simulink model "SistemaNL"  (R2026a)
settings: Solver=VariableStepAuto
settings Model: Creator=admin  LastModifiedBy=admin

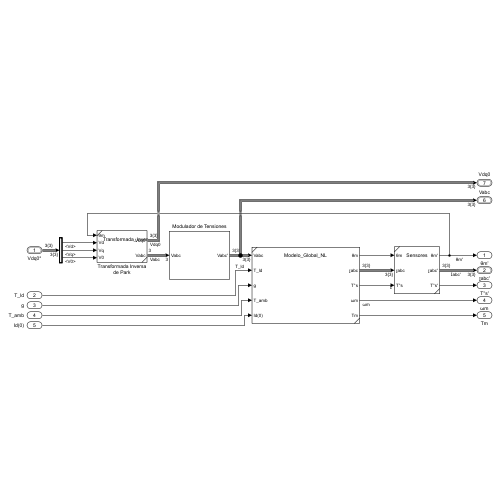
[thumbnail: Simulink's stored preview of the top-level diagram]
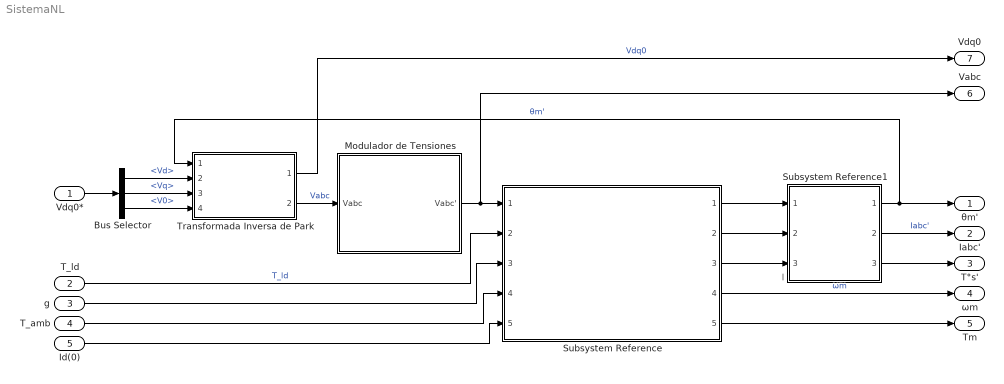
== system SistemaNL ==
  note: Ⅰ
  Vdq0* : Inport  OutDataTypeStr=Bus: Vdq0
  T_ld : Inport  Port=2
  g : Inport  Port=3
  T_amb : Inport  Port=4
  Id(0) : Inport  Port=5
  Bus Selector : BusSelector  OutputSignals=Vd,Vq,V0
  Modulador de Tensiones : Subsystem
  Subsystem Reference : Subsystem  ReferencedSubsystem=Modelo_Global_NL
  Subsystem Reference1 : Subsystem  ReferencedSubsystem=Sensores
  Transformada Inversa de Park : Subsystem  ReferencedSubsystem=Transformada_Inversa_de_Park_V
  θm' : Outport
  Ⅰabc' : Outport  Port=2  OutDataTypeStr=Bus: Iabc
  T°s' : Outport  Port=3
  ωm : Outport  Port=4
  Tm : Outport  Port=5
  Vabc : Outport  Port=6  OutDataTypeStr=Bus: Vabc
  Vdq0 : Outport  Port=7  OutDataTypeStr=Bus: Vdq0
  wires:
  Subsystem Reference1/2 -> Ⅰabc'/1  "Ⅰabc'"
  Subsystem Reference1/1 -> Transformada Inversa de Park/1, θm'/1  "θm'"
  Subsystem Reference1/3 -> T°s'/1
  Subsystem Reference/5 -> Tm/1
  Subsystem Reference/2 -> Subsystem Reference1/2
  g/1 -> Subsystem Reference/3
  Modulador de Tensiones/1(Vabc') -> Vabc/1, Subsystem Reference/1
  Subsystem Reference/4 -> ωm/1  "ωm"
  Subsystem Reference/1 -> Subsystem Reference1/1
  Subsystem Reference/3 -> Subsystem Reference1/3
  Transformada Inversa de Park/2 -> Modulador de Tensiones/1(Vabc)  "Vabc"
  T_ld/1 -> Subsystem Reference/2  "T_ld"
  Vdq0*/1 -> Bus Selector/1
  T_amb/1 -> Subsystem Reference/4
  Bus Selector/1 -> Transformada Inversa de Park/2  "<Vd>"
  Bus Selector/2 -> Transformada Inversa de Park/3  "<Vq>"
  Bus Selector/3 -> Transformada Inversa de Park/4  "<V0>"
  Transformada Inversa de Park/1 -> Vdq0/1  "Vdq0"
  Id(0)/1 -> Subsystem Reference/5

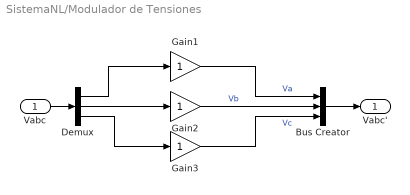
== system SistemaNL/Modulador de Tensiones ==
  Vabc : Inport
  Bus Creator : BusCreator  Inputs=3
  Demux : Demux  Outputs=3
  Gain1 : Gain
  Gain2 : Gain
  Gain3 : Gain
  Vabc' : Outport
  wires:
  Gain2/1 -> Bus Creator/2  "Vb"
  Gain3/1 -> Bus Creator/3  "Vc"
  Gain1/1 -> Bus Creator/1  "Va"
  Demux/2 -> Gain2/1
  Vabc/1 -> Demux/1
  Demux/1 -> Gain1/1
  Demux/3 -> Gain3/1
  Bus Creator/1 -> Vabc'/1
